simulink model "main"  (R2019b)
settings: Solver=VariableStepAuto  StartTime=0.0  StopTime=0.19  FixedStep=2e-4  RelTol=1e-3
values from neighbouring files (symbols this model uses):
  accCoef = 25    [RunSim.m]
  jerkCoef = 0.0090    (= 0.009)    [RunSim.m]
  snapCoef = 2.415e-6 + 4.5094e-07    (= 2.86594e-06)    [RunSim.m]
  Ts = 1/fs    (= 0.0002)    [initSim.m]
libraries: cstblocks x2, simulink x1, dspfdesign x1, model_controller x1
settings Model: Creator=Dai Luyao  LastModifiedBy=Princess
settings DataIOCC: ReturnWorkspaceOutputs=off
settings DebuggingCC: ArithmeticOperatorsInVariantConditions=warning
settings SFSimCC: SimUseLocalCustomCode=off  CustomCodeUndefinedFunction=UseInterfaceOnly
settings RTWCC: RTWUseLocalCustomCode=off
settings CodeAppCC: StateflowObjectComments=on

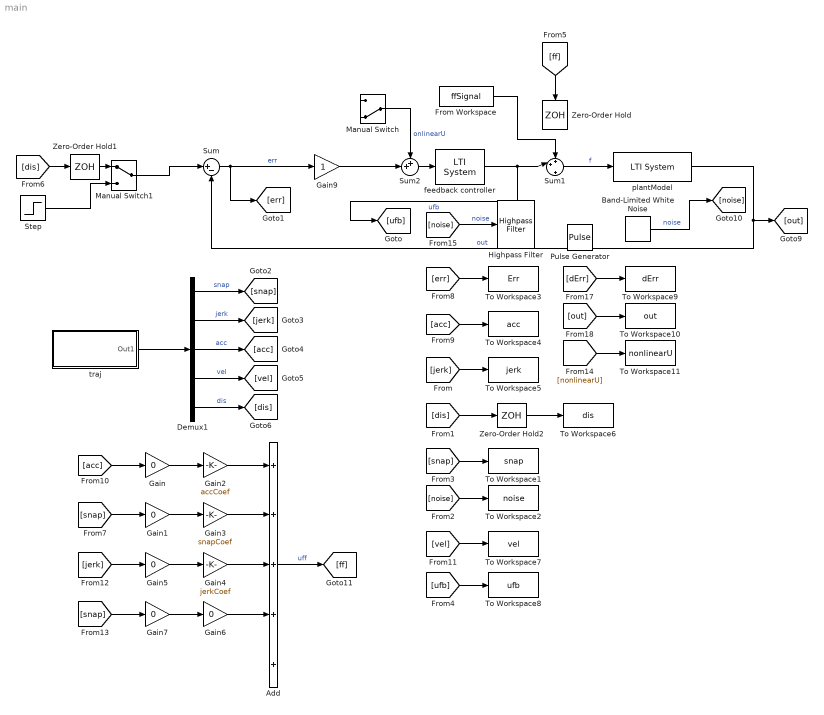
== system main ==
  Add : Sum  Inputs=+++++
  Band-Limited White Noise : simulink/Sources/Band-Limited White Noise  Cov=noisePower  Ts=Ts  seed=[2331]
  Demux1 : Demux  Outputs=5
  From Workspace : FromWorkspace  VariableName=ffSignal  SampleTime=Ts
  Gain{,1,5..7} (5 alike) : Gain  Gain=0
  Gain2 : Gain  Gain=accCoef
  Gain3 : Gain  Gain=snapCoef
  Gain4 : Gain  Gain=jerkCoef
  Gain9 : Gain
  Highpass Filter : dspfdesign/Highpass Filter  FilterType=IIR  DesignForMinimumOrder=off  FilterOrder=4  StopbandFrequency=8e3  PassbandFrequency=400  StopbandAttenuation=80  PassbandRipple=1  InheritSampleRate=off  SampleRate=5000  SimulateUsing=Interpreted execution  roundingMode=Floor  coeffsDataTypeStr=fixdt(1,16)
      settings: SourceProductName=DSP System Toolbox
  Manual Switch : ManualSwitch  CurrentSetting=0
  Manual Switch1 : ManualSwitch
  Pulse Generator : DiscretePulseGenerator  PulseType=Time based  Amplitude=10  Period=0.01  PulseWidth=5
  Step : Step  Time=0  After=30e-6  SampleTime=0
  Sum : Sum  Inputs=|+-
  Sum1 : Sum  Inputs=++|+
  Sum2 : Sum  Inputs=++|
  To Workspace1 : ToWorkspace  VariableName=snap  SaveFormat=Structure With Time  SampleTime=Ts
  To Workspace10 : ToWorkspace  VariableName=out  SaveFormat=Structure With Time  SampleTime=Ts
  To Workspace11 : ToWorkspace  VariableName=nonlinearU  SaveFormat=Structure With Time  SampleTime=Ts
  To Workspace2 : ToWorkspace  VariableName=noise  SaveFormat=Structure With Time  SampleTime=Ts
  To Workspace3 : ToWorkspace  VariableName=Err  SaveFormat=Structure With Time  SampleTime=Ts
  To Workspace4 : ToWorkspace  VariableName=acc  SaveFormat=Structure With Time  SampleTime=Ts
  To Workspace5 : ToWorkspace  VariableName=jerk  SaveFormat=Structure With Time  SampleTime=Ts
  To Workspace6 : ToWorkspace  VariableName=dis  SaveFormat=Structure With Time  SampleTime=Ts
  To Workspace7 : ToWorkspace  VariableName=vel  SaveFormat=Structure With Time  SampleTime=Ts
  To Workspace8 : ToWorkspace  VariableName=ufb  SaveFormat=Structure With Time  SampleTime=Ts
  To Workspace9 : ToWorkspace  VariableName=dErr  SaveFormat=Structure With Time  SampleTime=Ts
  Zero-Order Hold : ZeroOrderHold  SampleTime=Ts
  Zero-Order Hold1 : ZeroOrderHold  SampleTime=Ts
  Zero-Order Hold2 : ZeroOrderHold  SampleTime=Ts
  feedback controller : cstblocks/LTI System  sys=GcDis  IC=[]
  plantModel : cstblocks/LTI System  sys=GpDis3  IC=[]
  traj : Subsystem  BlockChoice=4th order traj
      link override 2nd order traj: x=0.6  v=0.25  a=10
      link override 3rd order traj: j=trajParameters.jerk  v=trajParameters.vel  x=trajParameters.dis  a=trajParameters.acc
      link override 4th order traj: a=20  v=0.5  x=0.05  j=2000  d=1.5e6  Ts=Ts  t0=0.02
      link override step: vf=1e-6
      settings: AttributesFormatString=%<BlockChoice>  TemplateBlock=model_controller/Profile Generators/traj  MemberBlocks=2th order traj,3rd order traj,4th order traj,step
  wires:
  Sum/1 -> Gain9/1, [err]  "err"
  Demux1/1 -> [snap]  "snap"
  Demux1/2 -> [jerk]  "jerk"
  Demux1/3 -> [acc]  "acc"
  Demux1/4 -> [vel]  "vel"
  Demux1/5 -> [dis]  "dis"
  [acc] -> To Workspace4/1
  [acc] -> Gain/1
  [jerk] -> To Workspace5/1
  [dis] -> Zero-Order Hold2/1
  [err] -> To Workspace3/1
  [noise] -> To Workspace2/1
  [ff] -> Zero-Order Hold/1
  [snap] -> To Workspace1/1
  [snap] -> Gain1/1
  Gain/1 -> Gain2/1
  Gain1/1 -> Gain3/1
  Add/1 -> [ff]  "uff"
  Gain2/1 -> Add/1
  Gain3/1 -> Add/2
  [vel] -> To Workspace7/1
  Gain4/1 -> Add/3
  [jerk] -> Gain5/1
  Gain5/1 -> Gain4/1
  Gain7/1 -> Gain6/1
  [snap] -> Gain7/1
  Gain6/1 -> Add/4
  plantModel/1 -> [out], Sum/2  "out"
  traj/1(Out1) -> Demux1/1
  feedback controller/1 -> [ufb], Sum1/2  "ufb"
  Sum1/1 -> plantModel/1  "f"
  [ufb] -> To Workspace8/1
  Sum2/1 -> feedback controller/1
  Manual Switch/1 -> Sum2/1  "onlinearU"
  [dis] -> Zero-Order Hold1/1
  Step/1 -> Manual Switch1/2
  Zero-Order Hold1/1 -> Manual Switch1/1
  Band-Limited White Noise/1 -> [noise]  "noise"
  [dErr] -> To Workspace9/1
  [out] -> To Workspace10/1
  Gain9/1 -> Sum2/2
  [nonlinearU] -> To Workspace11/1
  Manual Switch1/1 -> Sum/1
  [noise] -> Highpass Filter/1  "noise"
  Zero-Order Hold2/1 -> To Workspace6/1
  From Workspace/1 -> Sum1/1

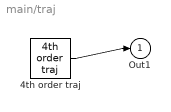
== system main/traj ==
  4th order traj : model_controller/Profile Generators/4th order traj  t0=0.02  x=0.05  v=0.5  a=20  j=2000  d=1.5e6  Ts=Ts
  Out1 : Outport
  wires:
  4th order traj/1 -> Out1/1
